simulink model "GPS_Constellation"  (R2018a)
settings: Solver=ode4  StartTime=0  StopTime=time_end  FixedStep=time_step  RelTol=1e-15  AbsTol=1e-15
values from neighbouring files (symbols this model uses):
  c = 299792458    [FFNAV_GPS_Params.mat]    (also in FFNAV_RunGPS.m; Test_GPS_Relativistic.m; Test_Klobuchar_Paper.m)
  GPS_COE = [4.6796815102 2.82369838363 0.203784643463 0.729652347089 1.65659671282 1.15813067845 3.02528391224 5.41010180216 3.56703411206 1.95260455396 0.205879038565 5.92829005708 ... (162 elements, 27x6)]    [FFNAV_GPS_Params.mat]    (also in FFNAV_RunGPS.m = [  268.126*deg2rad    SMA_GPS   ECC_GPS   INC_GPS   357.734*)
  mu = 398600441800000    [FFNAV_GPS_Params.mat]    (also in FFNAV_RunGPS.m; Test_GPS_Relativistic.m = 398600500000000)
undefined symbols (not defined in the file or in its folder): COE_chaser, COE_target
libraries: dspmtrx3 x27
(part 1 of 3)
settings Model: Creator=Cory  LastModifiedBy=Cory
settings SolverCC: AutoScaleAbsTol=off

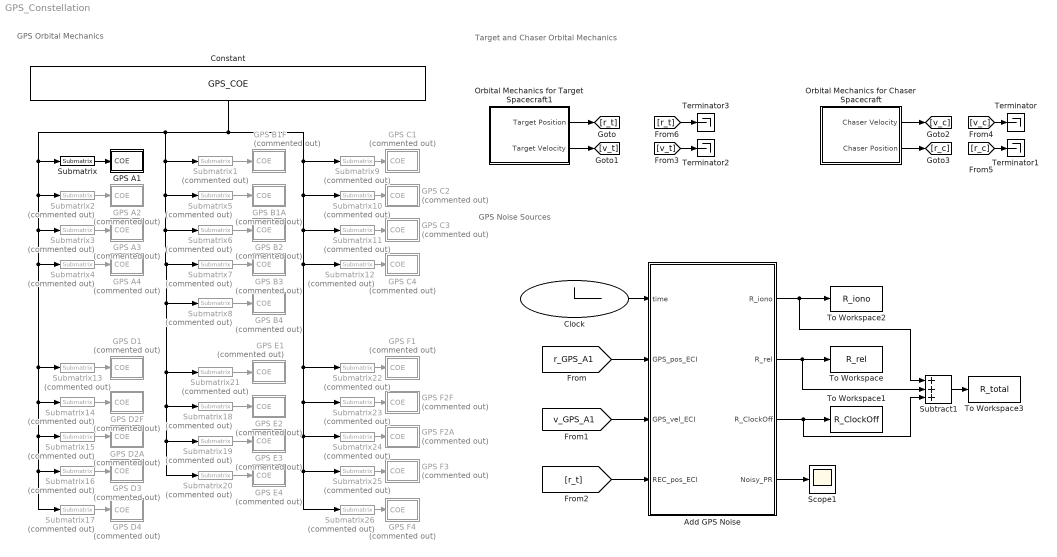
== system GPS_Constellation ==
  note: GPS Noise Sources
  note: GPS Orbital Mechanics
  note: Target and Chaser Orbital Mechanics
  Add GPS Noise : MATLAB Function  TreatAsAtomicUnit=on
  Clock : Clock
      settings: Decimation=1000
  Constant : Constant  Value=GPS_COE
  "GPS A1 " : Subsystem
      mask Display: image('C:\Users\Cory\OneDrive\FFNAV Project\MATLAB Code\NERM EKF Simulation\Masks\GPS Image.jpg');
  GPS A2 : Subsystem  Commented=on
      mask Display: image('C:\Users\Cory\OneDrive\FFNAV Project\MATLAB Code\NERM EKF Simulation\Masks\GPS Image.jpg');
  GPS A3 : Subsystem  Commented=on
      mask Display: image('C:\Users\Cory\OneDrive\FFNAV Project\MATLAB Code\NERM EKF Simulation\Masks\GPS Image.jpg');
  GPS A4 : Subsystem  Commented=on
      mask Display: image('C:\Users\Cory\OneDrive\FFNAV Project\MATLAB Code\NERM EKF Simulation\Masks\GPS Image.jpg');
  GPS B1A : Subsystem  Commented=on
      mask Display: image('C:\Users\Cory\OneDrive\FFNAV Project\MATLAB Code\NERM EKF Simulation\Masks\GPS Image.jpg');
  GPS B1F : Subsystem  Commented=on
      mask Display: image('C:\Users\Cory\OneDrive\FFNAV Project\MATLAB Code\NERM EKF Simulation\Masks\GPS Image.jpg');
  GPS B2 : Subsystem  Commented=on
      mask Display: image('C:\Users\Cory\OneDrive\FFNAV Project\MATLAB Code\NERM EKF Simulation\Masks\GPS Image.jpg');
  GPS B3 : Subsystem  Commented=on
      mask Display: image('C:\Users\Cory\OneDrive\FFNAV Project\MATLAB Code\NERM EKF Simulation\Masks\GPS Image.jpg');
  GPS B4 : Subsystem  Commented=on
      mask Display: image('C:\Users\Cory\OneDrive\FFNAV Project\MATLAB Code\NERM EKF Simulation\Masks\GPS Image.jpg');
  GPS C1 : Subsystem  Commented=on
      mask Display: image('C:\Users\Cory\OneDrive\FFNAV Project\MATLAB Code\NERM EKF Simulation\Masks\GPS Image.jpg');
  GPS C2 : Subsystem  Commented=on
      mask Display: image('C:\Users\Cory\OneDrive\FFNAV Project\MATLAB Code\NERM EKF Simulation\Masks\GPS Image.jpg');
  GPS C3 : Subsystem  Commented=on
      mask Display: image('C:\Users\Cory\OneDrive\FFNAV Project\MATLAB Code\NERM EKF Simulation\Masks\GPS Image.jpg');
  GPS C4 : Subsystem  Commented=on
      mask Display: image('C:\Users\Cory\OneDrive\FFNAV Project\MATLAB Code\NERM EKF Simulation\Masks\GPS Image.jpg');
  GPS D1 : Subsystem  Commented=on
      mask Display: image('C:\Users\Cory\OneDrive\FFNAV Project\MATLAB Code\NERM EKF Simulation\Masks\GPS Image.jpg');
  GPS D2A : Subsystem  Commented=on
      mask Display: image('C:\Users\Cory\OneDrive\FFNAV Project\MATLAB Code\NERM EKF Simulation\Masks\GPS Image.jpg');
  GPS D2F : Subsystem  Commented=on
      mask Display: image('C:\Users\Cory\OneDrive\FFNAV Project\MATLAB Code\NERM EKF Simulation\Masks\GPS Image.jpg');
  GPS D3 : Subsystem  Commented=on
      mask Display: image('C:\Users\Cory\OneDrive\FFNAV Project\MATLAB Code\NERM EKF Simulation\Masks\GPS Image.jpg');
  GPS D4 : Subsystem  Commented=on
      mask Display: image('C:\Users\Cory\OneDrive\FFNAV Project\MATLAB Code\NERM EKF Simulation\Masks\GPS Image.jpg');
  GPS E1 : Subsystem  Commented=on
      mask Display: image('C:\Users\Cory\OneDrive\FFNAV Project\MATLAB Code\NERM EKF Simulation\Masks\GPS Image.jpg');
  GPS E2 : Subsystem  Commented=on
      mask Display: image('C:\Users\Cory\OneDrive\FFNAV Project\MATLAB Code\NERM EKF Simulation\Masks\GPS Image.jpg');
  GPS E3 : Subsystem  Commented=on
      mask Display: image('C:\Users\Cory\OneDrive\FFNAV Project\MATLAB Code\NERM EKF Simulation\Masks\GPS Image.jpg');
  GPS E4 : Subsystem  Commented=on
      mask Display: image('C:\Users\Cory\OneDrive\FFNAV Project\MATLAB Code\NERM EKF Simulation\Masks\GPS Image.jpg');
  GPS F1 : Subsystem  Commented=on
      mask Display: image('C:\Users\Cory\OneDrive\FFNAV Project\MATLAB Code\NERM EKF Simulation\Masks\GPS Image.jpg');
  GPS F2A : Subsystem  Commented=on
      mask Display: image('C:\Users\Cory\OneDrive\FFNAV Project\MATLAB Code\NERM EKF Simulation\Masks\GPS Image.jpg');
  GPS F2F : Subsystem  Commented=on
      mask Display: image('C:\Users\Cory\OneDrive\FFNAV Project\MATLAB Code\NERM EKF Simulation\Masks\GPS Image.jpg');
  GPS F3 : Subsystem  Commented=on
      mask Display: image('C:\Users\Cory\OneDrive\FFNAV Project\MATLAB Code\NERM EKF Simulation\Masks\GPS Image.jpg');
  GPS F4 : Subsystem  Commented=on
      mask Display: image('C:\Users\Cory\OneDrive\FFNAV Project\MATLAB Code\NERM EKF Simulation\Masks\GPS Image.jpg');
  Orbital Mechanics for Target Spacecraft1 : Subsystem
  Orbital Mechanics for Chaser Spacecraft : Subsystem
  Scope1 : Scope
  Submatrix : dspmtrx3/Submatrix  RowSpan=One row  RowStartMode=Index  RowStartIndex=1  RowEndMode=Last  RowEndIndex=1  ColSpan=All columns  ColStartMode=First  ColStartIndex=1  ColEndMode=Last  ColEndIndex=1
  Submatrix1 : dspmtrx3/Submatrix  Commented=on  RowSpan=One row  RowStartMode=Index  RowStartIndex=5  RowEndMode=Last  RowEndIndex=1  ColSpan=All columns  ColStartMode=First  ColStartIndex=1  ColEndMode=Last  ColEndIndex=1
  Submatrix10 : dspmtrx3/Submatrix  Commented=on  RowSpan=One row  RowStartMode=Index  RowStartIndex=11  RowEndMode=Last  RowEndIndex=1  ColSpan=All columns  ColStartMode=First  ColStartIndex=1  ColEndMode=Last  ColEndIndex=1
  Submatrix11 : dspmtrx3/Submatrix  Commented=on  RowSpan=One row  RowStartMode=Index  RowStartIndex=12  RowEndMode=Last  RowEndIndex=1  ColSpan=All columns  ColStartMode=First  ColStartIndex=1  ColEndMode=Last  ColEndIndex=1
  Submatrix12 : dspmtrx3/Submatrix  Commented=on  RowSpan=One row  RowStartMode=Index  RowStartIndex=13  RowEndMode=Last  RowEndIndex=1  ColSpan=All columns  ColStartMode=First  ColStartIndex=1  ColEndMode=Last  ColEndIndex=1
  Submatrix13 : dspmtrx3/Submatrix  Commented=on  RowSpan=One row  RowStartMode=Index  RowStartIndex=14  RowEndMode=Last  RowEndIndex=1  ColSpan=All columns  ColStartMode=First  ColStartIndex=1  ColEndMode=Last  ColEndIndex=1
  Submatrix14 : dspmtrx3/Submatrix  Commented=on  RowSpan=One row  RowStartMode=Index  RowStartIndex=15  RowEndMode=Last  RowEndIndex=1  ColSpan=All columns  ColStartMode=First  ColStartIndex=1  ColEndMode=Last  ColEndIndex=1
  Submatrix15 : dspmtrx3/Submatrix  Commented=on  RowSpan=One row  RowStartMode=Index  RowStartIndex=16  RowEndMode=Last  RowEndIndex=1  ColSpan=All columns  ColStartMode=First  ColStartIndex=1  ColEndMode=Last  ColEndIndex=1
  Submatrix16 : dspmtrx3/Submatrix  Commented=on  RowSpan=One row  RowStartMode=Index  RowStartIndex=17  RowEndMode=Last  RowEndIndex=1  ColSpan=All columns  ColStartMode=First  ColStartIndex=1  ColEndMode=Last  ColEndIndex=1
  Submatrix17 : dspmtrx3/Submatrix  Commented=on  RowSpan=One row  RowStartMode=Index  RowStartIndex=18  RowEndMode=Last  RowEndIndex=1  ColSpan=All columns  ColStartMode=First  ColStartIndex=1  ColEndMode=Last  ColEndIndex=1
  Submatrix18 : dspmtrx3/Submatrix  Commented=on  RowSpan=One row  RowStartMode=Index  RowStartIndex=20  RowEndMode=Last  RowEndIndex=1  ColSpan=All columns  ColStartMode=First  ColStartIndex=1  ColEndMode=Last  ColEndIndex=1
  Submatrix19 : dspmtrx3/Submatrix  Commented=on  RowSpan=One row  RowStartMode=Index  RowStartIndex=21  RowEndMode=Last  RowEndIndex=1  ColSpan=All columns  ColStartMode=First  ColStartIndex=1  ColEndMode=Last  ColEndIndex=1
  Submatrix2 : dspmtrx3/Submatrix  Commented=on  RowSpan=One row  RowStartMode=Index  RowStartIndex=2  RowEndMode=Last  RowEndIndex=1  ColSpan=All columns  ColStartMode=First  ColStartIndex=1  ColEndMode=Last  ColEndIndex=1
  Submatrix20 : dspmtrx3/Submatrix  Commented=on  RowSpan=One row  RowStartMode=Index  RowStartIndex=22  RowEndMode=Last  RowEndIndex=1  ColSpan=All columns  ColStartMode=First  ColStartIndex=1  ColEndMode=Last  ColEndIndex=1
  Submatrix21 : dspmtrx3/Submatrix  Commented=on  RowSpan=One row  RowStartMode=Index  RowStartIndex=19  RowEndMode=Last  RowEndIndex=1  ColSpan=All columns  ColStartMode=First  ColStartIndex=1  ColEndMode=Last  ColEndIndex=1
  Submatrix22 : dspmtrx3/Submatrix  Commented=on  RowSpan=One row  RowStartMode=Index  RowStartIndex=23  RowEndMode=Last  RowEndIndex=1  ColSpan=All columns  ColStartMode=First  ColStartIndex=1  ColEndMode=Last  ColEndIndex=1
  Submatrix23 : dspmtrx3/Submatrix  Commented=on  RowSpan=One row  RowStartMode=Index  RowStartIndex=24  RowEndMode=Last  RowEndIndex=1  ColSpan=All columns  ColStartMode=First  ColStartIndex=1  ColEndMode=Last  ColEndIndex=1
  Submatrix24 : dspmtrx3/Submatrix  Commented=on  RowSpan=One row  RowStartMode=Index  RowStartIndex=25  RowEndMode=Last  RowEndIndex=1  ColSpan=All columns  ColStartMode=First  ColStartIndex=1  ColEndMode=Last  ColEndIndex=1
  Submatrix25 : dspmtrx3/Submatrix  Commented=on  RowSpan=One row  RowStartMode=Index  RowStartIndex=26  RowEndMode=Last  RowEndIndex=1  ColSpan=All columns  ColStartMode=First  ColStartIndex=1  ColEndMode=Last  ColEndIndex=1
  Submatrix26 : dspmtrx3/Submatrix  Commented=on  RowSpan=One row  RowStartMode=Index  RowStartIndex=27  RowEndMode=Last  RowEndIndex=1  ColSpan=All columns  ColStartMode=First  ColStartIndex=1  ColEndMode=Last  ColEndIndex=1
  Submatrix3 : dspmtrx3/Submatrix  Commented=on  RowSpan=One row  RowStartMode=Index  RowStartIndex=3  RowEndMode=Last  RowEndIndex=1  ColSpan=All columns  ColStartMode=First  ColStartIndex=1  ColEndMode=Last  ColEndIndex=1
  Submatrix4 : dspmtrx3/Submatrix  Commented=on  RowSpan=One row  RowStartMode=Index  RowStartIndex=4  RowEndMode=Last  RowEndIndex=1  ColSpan=All columns  ColStartMode=First  ColStartIndex=1  ColEndMode=Last  ColEndIndex=1
  Submatrix5 : dspmtrx3/Submatrix  Commented=on  RowSpan=One row  RowStartMode=Index  RowStartIndex=6  RowEndMode=Last  RowEndIndex=1  ColSpan=All columns  ColStartMode=First  ColStartIndex=1  ColEndMode=Last  ColEndIndex=1
  Submatrix6 : dspmtrx3/Submatrix  Commented=on  RowSpan=One row  RowStartMode=Index  RowStartIndex=7  RowEndMode=Last  RowEndIndex=1  ColSpan=All columns  ColStartMode=First  ColStartIndex=1  ColEndMode=Last  ColEndIndex=1
  Submatrix7 : dspmtrx3/Submatrix  Commented=on  RowSpan=One row  RowStartMode=Index  RowStartIndex=8  RowEndMode=Last  RowEndIndex=1  ColSpan=All columns  ColStartMode=First  ColStartIndex=1  ColEndMode=Last  ColEndIndex=1
  Submatrix8 : dspmtrx3/Submatrix  Commented=on  RowSpan=One row  RowStartMode=Index  RowStartIndex=9  RowEndMode=Last  RowEndIndex=1  ColSpan=All columns  ColStartMode=First  ColStartIndex=1  ColEndMode=Last  ColEndIndex=1
  Submatrix9 : dspmtrx3/Submatrix  Commented=on  RowSpan=One row  RowStartMode=Index  RowStartIndex=10  RowEndMode=Last  RowEndIndex=1  ColSpan=All columns  ColStartMode=First  ColStartIndex=1  ColEndMode=Last  ColEndIndex=1
  Subtract1 : Sum  Inputs=+++
  Terminator{,1..3} (4 alike) : Terminator
  To Workspace : ToWorkspace  VariableName=R_rel  SampleTime=-1
      settings: Save2DSignal=2-D array (concatenate along first dimension)
  To Workspace1 : ToWorkspace  VariableName=R_ClockOff  SampleTime=-1
      settings: Save2DSignal=2-D array (concatenate along first dimension)
  To Workspace2 : ToWorkspace  VariableName=R_iono  SampleTime=-1
      settings: Save2DSignal=2-D array (concatenate along first dimension)
  To Workspace3 : ToWorkspace  VariableName=R_total  SampleTime=-1
      settings: Save2DSignal=2-D array (concatenate along first dimension)
  wires:
  Submatrix/1 -> "GPS A1 "/1(COE)
  Submatrix1/1 -> GPS B1F/1(COE)
  Submatrix2/1 -> GPS A2/1(COE)
  Submatrix3/1 -> GPS A3/1(COE)
  Submatrix4/1 -> GPS A4/1(COE)
  Submatrix5/1 -> GPS B1A/1(COE)
  Submatrix6/1 -> GPS B2/1(COE)
  Submatrix7/1 -> GPS B3/1(COE)
  Submatrix8/1 -> GPS B4/1(COE)
  Submatrix10/1 -> GPS C2/1(COE)
  Submatrix11/1 -> GPS C3/1(COE)
  Submatrix12/1 -> GPS C4/1(COE)
  Submatrix9/1 -> GPS C1/1(COE)
  Submatrix14/1 -> GPS D2F/1(COE)
  Submatrix15/1 -> GPS D2A/1(COE)
  Submatrix17/1 -> GPS D4/1(COE)
  Submatrix16/1 -> GPS D3/1(COE)
  Submatrix13/1 -> GPS D1/1(COE)
  Submatrix19/1 -> GPS E3/1(COE)
  Submatrix18/1 -> GPS E2/1(COE)
  Submatrix21/1 -> GPS E1/1(COE)
  Submatrix20/1 -> GPS E4/1(COE)
  Submatrix23/1 -> GPS F2F/1(COE)
  Constant/1 -> Submatrix17/1, Submatrix16/1, Submatrix15/1, Submatrix14/1, Submatrix13/1, Submatrix4/1, Submatrix3/1, Submatrix2/1, Submatrix/1, Submatrix8/1, Submatrix21/1, Submatrix18/1, Submatrix19/1, Submatrix20/1, Submatrix7/1, Submatrix6/1, Submatrix5/1, Submatrix1/1, Submatrix12/1, Submatrix22/1, Submatrix23/1, Submatrix24/1, Submatrix25/1, Submatrix26/1, Submatrix11/1, Submatrix10/1, Submatrix9/1
  Submatrix26/1 -> GPS F4/1(COE)
  Submatrix24/1 -> GPS F2A/1(COE)
  Submatrix25/1 -> GPS F3/1(COE)
  Submatrix22/1 -> GPS F1/1(COE)
  Clock/1 -> Add GPS Noise/1(time)
  Add GPS Noise/1(R_iono) -> Subtract1/1, To Workspace2/1
  Add GPS Noise/4(Noisy_PR) -> Scope1/1
  [r_GPS_A1] -> Add GPS Noise/2(GPS_pos_ECI)
  [v_GPS_A1] -> Add GPS Noise/3(GPS_vel_ECI)
  [r_t] -> Add GPS Noise/4(REC_pos_ECI)
  Add GPS Noise/2(R_rel) -> Subtract1/2, To Workspace/1
  Add GPS Noise/3(R_ClockOff) -> Subtract1/3, To Workspace1/1
  Subtract1/1 -> To Workspace3/1
  Orbital Mechanics for Chaser Spacecraft/2(Chaser Position) -> [r_c]
  Orbital Mechanics for Target Spacecraft1/1(Target Position) -> [r_t]
  Orbital Mechanics for Target Spacecraft1/2(Target Velocity) -> [v_t]
  Orbital Mechanics for Chaser Spacecraft/1(Chaser Velocity) -> [v_c]
  [v_c] -> Terminator/1
  [r_c] -> Terminator1/1
  [v_t] -> Terminator2/1
  [r_t] -> Terminator3/1

== system GPS_Constellation/GPS A1  ==
  COE : Inport
  Mux : Mux  Inputs=2
  Orbital Mechanics : Subsystem
  To Workspace : ToWorkspace  VariableName=GPS_A1  SampleTime=-1
      settings: Save2DSignal=2-D array (concatenate along first dimension)
  tag scope: r_GPS_A1=global, v_GPS_A1=global
  wires:
  Orbital Mechanics/2(Velocity (v)) -> [v_GPS_A1], Mux/2
  COE/1 -> Orbital Mechanics/1(COE)
  Mux/1 -> To Workspace/1
  Orbital Mechanics/1(Position (r)) -> Mux/1, [r_GPS_A1]

== system GPS_Constellation/GPS A2 ==
  COE : Inport
  Mux : Mux  Inputs=2
  Orbital Mechanics1 : Subsystem
  To Workspace : ToWorkspace  VariableName=GPS_A2  SampleTime=-1
      settings: Save2DSignal=2-D array (concatenate along first dimension)
  wires:
  Orbital Mechanics1/2(Velocity (v)) -> Mux/2
  COE/1 -> Orbital Mechanics1/1(COE)
  Orbital Mechanics1/1(Position (r)) -> Mux/1
  Mux/1 -> To Workspace/1

== system GPS_Constellation/GPS A3 ==
  COE : Inport
  Mux : Mux  Inputs=2
  Orbital Mechanics : Subsystem
  To Workspace : ToWorkspace  VariableName=GPS_A3  SampleTime=-1
      settings: Save2DSignal=2-D array (concatenate along first dimension)
  wires:
  Orbital Mechanics/2(Velocity (v)) -> Mux/2
  COE/1 -> Orbital Mechanics/1(COE)
  Orbital Mechanics/1(Position (r)) -> Mux/1
  Mux/1 -> To Workspace/1

== system GPS_Constellation/GPS A4 ==
  COE : Inport
  Mux : Mux  Inputs=2
  Orbital Mechanics : Subsystem
  To Workspace : ToWorkspace  VariableName=GPS_A4  SampleTime=-1
      settings: Save2DSignal=2-D array (concatenate along first dimension)
  wires:
  Orbital Mechanics/2(Velocity (v)) -> Mux/2
  COE/1 -> Orbital Mechanics/1(COE)
  Orbital Mechanics/1(Position (r)) -> Mux/1
  Mux/1 -> To Workspace/1

== system GPS_Constellation/GPS B1A ==
  COE : Inport
  Mux : Mux  Inputs=2
  Orbital Mechanics : Subsystem
  To Workspace : ToWorkspace  VariableName=GPS_B1A  SampleTime=-1
      settings: Save2DSignal=2-D array (concatenate along first dimension)
  wires:
  Orbital Mechanics/2(Velocity (v)) -> Mux/2
  COE/1 -> Orbital Mechanics/1(COE)
  Orbital Mechanics/1(Position (r)) -> Mux/1
  Mux/1 -> To Workspace/1

== system GPS_Constellation/GPS B1F ==
  COE : Inport
  Mux : Mux  Inputs=2
  Orbital Mechanics : Subsystem
  To Workspace : ToWorkspace  VariableName=GPS_B1F  SampleTime=-1
      settings: Save2DSignal=2-D array (concatenate along first dimension)
  wires:
  Orbital Mechanics/2(Velocity (v)) -> Mux/2
  COE/1 -> Orbital Mechanics/1(COE)
  Orbital Mechanics/1(Position (r)) -> Mux/1
  Mux/1 -> To Workspace/1

== system GPS_Constellation/GPS B2 ==
  COE : Inport
  Mux : Mux  Inputs=2
  Orbital Mechanics : Subsystem
  To Workspace : ToWorkspace  VariableName=GPS_B2  SampleTime=-1
      settings: Save2DSignal=2-D array (concatenate along first dimension)
  wires:
  Orbital Mechanics/2(Velocity (v)) -> Mux/2
  COE/1 -> Orbital Mechanics/1(COE)
  Orbital Mechanics/1(Position (r)) -> Mux/1
  Mux/1 -> To Workspace/1

== system GPS_Constellation/GPS B3 ==
  COE : Inport
  Mux : Mux  Inputs=2
  Orbital Mechanics : Subsystem
  To Workspace : ToWorkspace  VariableName=GPS_B3  SampleTime=-1
      settings: Save2DSignal=2-D array (concatenate along first dimension)
  wires:
  Orbital Mechanics/2(Velocity (v)) -> Mux/2
  COE/1 -> Orbital Mechanics/1(COE)
  Orbital Mechanics/1(Position (r)) -> Mux/1
  Mux/1 -> To Workspace/1

== system GPS_Constellation/GPS B4 ==
  COE : Inport
  Mux : Mux  Inputs=2
  Orbital Mechanics : Subsystem
  To Workspace : ToWorkspace  VariableName=GPS_B4  SampleTime=-1
      settings: Save2DSignal=2-D array (concatenate along first dimension)
  wires:
  Orbital Mechanics/2(Velocity (v)) -> Mux/2
  COE/1 -> Orbital Mechanics/1(COE)
  Orbital Mechanics/1(Position (r)) -> Mux/1
  Mux/1 -> To Workspace/1

== system GPS_Constellation/GPS C1 ==
  COE : Inport
  Mux : Mux  Inputs=2
  Orbital Mechanics : Subsystem
  To Workspace : ToWorkspace  VariableName=GPS_C1  SampleTime=-1
      settings: Save2DSignal=2-D array (concatenate along first dimension)
  wires:
  Orbital Mechanics/2(Velocity (v)) -> Mux/2
  COE/1 -> Orbital Mechanics/1(COE)
  Orbital Mechanics/1(Position (r)) -> Mux/1
  Mux/1 -> To Workspace/1

== system GPS_Constellation/GPS C2 ==
  COE : Inport
  Mux : Mux  Inputs=2
  Orbital Mechanics : Subsystem
  To Workspace : ToWorkspace  VariableName=GPS_C2  SampleTime=-1
      settings: Save2DSignal=2-D array (concatenate along first dimension)
  wires:
  Orbital Mechanics/2(Velocity (v)) -> Mux/2
  COE/1 -> Orbital Mechanics/1(COE)
  Orbital Mechanics/1(Position (r)) -> Mux/1
  Mux/1 -> To Workspace/1

== system GPS_Constellation/GPS C3 ==
  COE : Inport
  Mux : Mux  Inputs=2
  Orbital Mechanics : Subsystem
  To Workspace : ToWorkspace  VariableName=GPS_C3  SampleTime=-1
      settings: Save2DSignal=2-D array (concatenate along first dimension)
  wires:
  Orbital Mechanics/2(Velocity (v)) -> Mux/2
  COE/1 -> Orbital Mechanics/1(COE)
  Orbital Mechanics/1(Position (r)) -> Mux/1
  Mux/1 -> To Workspace/1

== system GPS_Constellation/GPS C4 ==
  COE : Inport
  Mux : Mux  Inputs=2
  Orbital Mechanics : Subsystem
  To Workspace : ToWorkspace  VariableName=GPS_C4  SampleTime=-1
      settings: Save2DSignal=2-D array (concatenate along first dimension)
  wires:
  Orbital Mechanics/2(Velocity (v)) -> Mux/2
  COE/1 -> Orbital Mechanics/1(COE)
  Orbital Mechanics/1(Position (r)) -> Mux/1
  Mux/1 -> To Workspace/1

== system GPS_Constellation/GPS D1 ==
  COE : Inport
  Mux : Mux  Inputs=2
  Orbital Mechanics : Subsystem
  To Workspace : ToWorkspace  VariableName=GPS_D1  SampleTime=-1
      settings: Save2DSignal=2-D array (concatenate along first dimension)
  wires:
  Orbital Mechanics/2(Velocity (v)) -> Mux/2
  COE/1 -> Orbital Mechanics/1(COE)
  Orbital Mechanics/1(Position (r)) -> Mux/1
  Mux/1 -> To Workspace/1

== system GPS_Constellation/GPS D2A ==
  COE : Inport
  Mux : Mux  Inputs=2
  Orbital Mechanics : Subsystem
  To Workspace : ToWorkspace  VariableName=GPS_D2A  SampleTime=-1
      settings: Save2DSignal=2-D array (concatenate along first dimension)
  wires:
  Orbital Mechanics/2(Velocity (v)) -> Mux/2
  COE/1 -> Orbital Mechanics/1(COE)
  Orbital Mechanics/1(Position (r)) -> Mux/1
  Mux/1 -> To Workspace/1

== system GPS_Constellation/GPS D2F ==
  COE : Inport
  Mux : Mux  Inputs=2
  Orbital Mechanics : Subsystem
  To Workspace : ToWorkspace  VariableName=GPS_D2F  SampleTime=-1
      settings: Save2DSignal=2-D array (concatenate along first dimension)
  wires:
  Orbital Mechanics/2(Velocity (v)) -> Mux/2
  COE/1 -> Orbital Mechanics/1(COE)
  Orbital Mechanics/1(Position (r)) -> Mux/1
  Mux/1 -> To Workspace/1

== system GPS_Constellation/GPS D3 ==
  COE : Inport
  Mux : Mux  Inputs=2
  Orbital Mechanics : Subsystem
  To Workspace : ToWorkspace  VariableName=GPS_D3  SampleTime=-1
      settings: Save2DSignal=2-D array (concatenate along first dimension)
  wires:
  Orbital Mechanics/2(Velocity (v)) -> Mux/2
  COE/1 -> Orbital Mechanics/1(COE)
  Orbital Mechanics/1(Position (r)) -> Mux/1
  Mux/1 -> To Workspace/1

== system GPS_Constellation/GPS D4 ==
  COE : Inport
  Mux : Mux  Inputs=2
  Orbital Mechanics : Subsystem
  To Workspace : ToWorkspace  VariableName=GPS_D4  SampleTime=-1
      settings: Save2DSignal=2-D array (concatenate along first dimension)
  wires:
  Orbital Mechanics/2(Velocity (v)) -> Mux/2
  COE/1 -> Orbital Mechanics/1(COE)
  Orbital Mechanics/1(Position (r)) -> Mux/1
  Mux/1 -> To Workspace/1

== system GPS_Constellation/GPS E1 ==
  COE : Inport
  Mux : Mux  Inputs=2
  Orbital Mechanics : Subsystem
  To Workspace : ToWorkspace  VariableName=GPS_E1  SampleTime=-1
      settings: Save2DSignal=2-D array (concatenate along first dimension)
  wires:
  Orbital Mechanics/2(Velocity (v)) -> Mux/2
  COE/1 -> Orbital Mechanics/1(COE)
  Orbital Mechanics/1(Position (r)) -> Mux/1
  Mux/1 -> To Workspace/1

== system GPS_Constellation/GPS E2 ==
  COE : Inport
  Mux : Mux  Inputs=2
  Orbital Mechanics : Subsystem
  To Workspace : ToWorkspace  VariableName=GPS_E2  SampleTime=-1
      settings: Save2DSignal=2-D array (concatenate along first dimension)
  wires:
  Orbital Mechanics/2(Velocity (v)) -> Mux/2
  COE/1 -> Orbital Mechanics/1(COE)
  Orbital Mechanics/1(Position (r)) -> Mux/1
  Mux/1 -> To Workspace/1

== system GPS_Constellation/GPS E3 ==
  COE : Inport
  Mux : Mux  Inputs=2
  Orbital Mechanics : Subsystem
  To Workspace : ToWorkspace  VariableName=GPS_E3  SampleTime=-1
      settings: Save2DSignal=2-D array (concatenate along first dimension)
  wires:
  Orbital Mechanics/2(Velocity (v)) -> Mux/2
  COE/1 -> Orbital Mechanics/1(COE)
  Orbital Mechanics/1(Position (r)) -> Mux/1
  Mux/1 -> To Workspace/1

== system GPS_Constellation/GPS E4 ==
  COE : Inport
  Mux : Mux  Inputs=2
  Orbital Mechanics : Subsystem
  To Workspace : ToWorkspace  VariableName=GPS_E4  SampleTime=-1
      settings: Save2DSignal=2-D array (concatenate along first dimension)
  wires:
  Orbital Mechanics/2(Velocity (v)) -> Mux/2
  COE/1 -> Orbital Mechanics/1(COE)
  Orbital Mechanics/1(Position (r)) -> Mux/1
  Mux/1 -> To Workspace/1

== system GPS_Constellation/GPS F1 ==
  COE : Inport
  Mux : Mux  Inputs=2
  Orbital Mechanics : Subsystem
  To Workspace : ToWorkspace  VariableName=GPS_F1  SampleTime=-1
      settings: Save2DSignal=2-D array (concatenate along first dimension)
  wires:
  Orbital Mechanics/2(Velocity (v)) -> Mux/2
  COE/1 -> Orbital Mechanics/1(COE)
  Orbital Mechanics/1(Position (r)) -> Mux/1
  Mux/1 -> To Workspace/1

== system GPS_Constellation/GPS F2A ==
  COE : Inport
  Mux : Mux  Inputs=2
  Orbital Mechanics : Subsystem
  To Workspace : ToWorkspace  VariableName=GPS_F2A  SampleTime=-1
      settings: Save2DSignal=2-D array (concatenate along first dimension)
  wires:
  Orbital Mechanics/2(Velocity (v)) -> Mux/2
  COE/1 -> Orbital Mechanics/1(COE)
  Orbital Mechanics/1(Position (r)) -> Mux/1
  Mux/1 -> To Workspace/1

== system GPS_Constellation/GPS F2F ==
  COE : Inport
  Mux : Mux  Inputs=2
  Orbital Mechanics : Subsystem
  To Workspace : ToWorkspace  VariableName=GPS_F2F  SampleTime=-1
      settings: Save2DSignal=2-D array (concatenate along first dimension)
  wires:
  Orbital Mechanics/2(Velocity (v)) -> Mux/2
  COE/1 -> Orbital Mechanics/1(COE)
  Orbital Mechanics/1(Position (r)) -> Mux/1
  Mux/1 -> To Workspace/1

== system GPS_Constellation/GPS F3 ==
  COE : Inport
  Mux : Mux  Inputs=2
  Orbital Mechanics : Subsystem
  To Workspace : ToWorkspace  VariableName=GPS_F3  SampleTime=-1
      settings: Save2DSignal=2-D array (concatenate along first dimension)
  wires:
  Orbital Mechanics/2(Velocity (v)) -> Mux/2
  COE/1 -> Orbital Mechanics/1(COE)
  Orbital Mechanics/1(Position (r)) -> Mux/1
  Mux/1 -> To Workspace/1

== system GPS_Constellation/GPS F4 ==
  COE : Inport
  Mux : Mux  Inputs=2
  Orbital Mechanics : Subsystem
  To Workspace : ToWorkspace  VariableName=GPS_F4  SampleTime=-1
      settings: Save2DSignal=2-D array (concatenate along first dimension)
  wires:
  Orbital Mechanics/2(Velocity (v)) -> Mux/2
  COE/1 -> Orbital Mechanics/1(COE)
  Orbital Mechanics/1(Position (r)) -> Mux/1
  Mux/1 -> To Workspace/1

== system GPS_Constellation/Orbital Mechanics for Target Spacecraft1 ==
  Integrator : Integrator  InitialConditionSource=external
  Integrator1 : Integrator  InitialConditionSource=external
  MATLAB Function1 : MATLAB Function  TreatAsAtomicUnit=on
  Target Orbital Mechanics : MATLAB Function  TreatAsAtomicUnit=on
  To Workspace1 : ToWorkspace  VariableName=r_target_ECI  SampleTime=-1
  To Workspace2 : ToWorkspace  VariableName=v_target_ECI  SampleTime=-1
  Target Position : Outport
  Target Velocity : Outport  Port=2
  wires:
  Integrator/1 -> To Workspace2/1, Target Velocity/1, Integrator1/1  "r_dot"
  MATLAB Function1/1(r_ddot) -> Integrator/1  "r_ddot"
  Integrator1/1 -> MATLAB Function1/1(r), To Workspace1/1, Target Position/1  "getr"
  Target Orbital Mechanics/2(r_ECI) -> Integrator1/2
  Target Orbital Mechanics/1(v_ECI) -> Integrator/2  "V0"

== system GPS_Constellation/Orbital Mechanics for Chaser Spacecraft ==
  Integrator : Integrator  InitialConditionSource=external
  Integrator1 : Integrator  InitialConditionSource=external
  MATLAB Function1 : MATLAB Function  TreatAsAtomicUnit=on
  Orbital Mechanics : MATLAB Function  TreatAsAtomicUnit=on
  To Workspace1 : ToWorkspace  VariableName=r_chaser_ECI  SampleTime=-1
  To Workspace2 : ToWorkspace  VariableName=v_chaser_ECI  SampleTime=-1
  Chaser Velocity : Outport
  Chaser Position : Outport  Port=2
  wires:
  Integrator/1 -> To Workspace2/1, Chaser Velocity/1, Integrator1/1  "r_dot"
  MATLAB Function1/1(r_ddot) -> Integrator/1  "r_ddot"
  Integrator1/1 -> To Workspace1/1, MATLAB Function1/1(r), Chaser Position/1  "r"
  Orbital Mechanics/2(r_ECI) -> Integrator1/2
  Orbital Mechanics/1(v_ECI) -> Integrator/2  "V0"

== system GPS_Constellation/GPS A1 /Orbital Mechanics ==
  COE : Inport
  Integrator : Integrator  InitialConditionSource=external
  Integrator1 : Integrator  InitialConditionSource=external
  MATLAB Function1 : MATLAB Function  TreatAsAtomicUnit=on
  Orbital Mechanics : MATLAB Function  TreatAsAtomicUnit=on
  Position (r) : Outport
  Velocity (v) : Outport  Port=2
  wires:
  Integrator/1 -> Velocity (v)/1, Integrator1/1  "r_dot"
  MATLAB Function1/1(r_ddot) -> Integrator/1  "r_ddot"
  Integrator1/1 -> Position (r)/1, MATLAB Function1/1(R_sat)  "r"
  Orbital Mechanics/2(r_ECI) -> Integrator1/2
  Orbital Mechanics/1(v_ECI) -> Integrator/2  "V0"
  COE/1 -> Orbital Mechanics/1(COE)

== system GPS_Constellation/GPS A2/Orbital Mechanics1 ==
  COE : Inport
  Integrator : Integrator  InitialConditionSource=external
  Integrator1 : Integrator  InitialConditionSource=external
  MATLAB Function1 : MATLAB Function  TreatAsAtomicUnit=on
  Orbital Mechanics : MATLAB Function  TreatAsAtomicUnit=on
  Position (r) : Outport
  Velocity (v) : Outport  Port=2
  wires:
  Integrator/1 -> Velocity (v)/1, Integrator1/1  "r_dot"
  MATLAB Function1/1(r_ddot) -> Integrator/1  "r_ddot"
  Integrator1/1 -> Position (r)/1, MATLAB Function1/1(r)  "r"
  Orbital Mechanics/2(r_ECI) -> Integrator1/2
  Orbital Mechanics/1(v_ECI) -> Integrator/2  "V0"
  COE/1 -> Orbital Mechanics/1(COE)

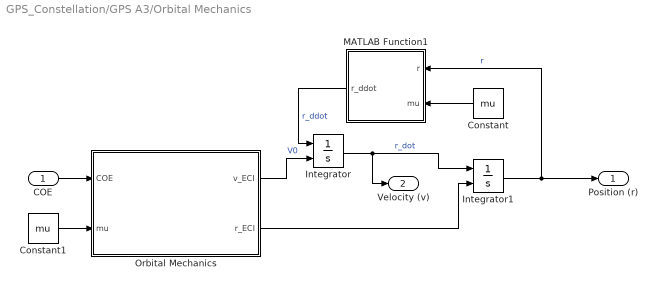
== system GPS_Constellation/GPS A3/Orbital Mechanics ==
  COE : Inport
  Constant : Constant  Value=mu
  Constant1 : Constant  Value=mu
  Integrator : Integrator  InitialConditionSource=external
  Integrator1 : Integrator  InitialConditionSource=external
  MATLAB Function1 : MATLAB Function  TreatAsAtomicUnit=on
  Orbital Mechanics : MATLAB Function  TreatAsAtomicUnit=on
  Position (r) : Outport
  Velocity (v) : Outport  Port=2
  wires:
  Integrator/1 -> Velocity (v)/1, Integrator1/1  "r_dot"
  MATLAB Function1/1(r_ddot) -> Integrator/1  "r_ddot"
  Integrator1/1 -> Position (r)/1, MATLAB Function1/1(r)  "r"
  Orbital Mechanics/2(r_ECI) -> Integrator1/2
  Orbital Mechanics/1(v_ECI) -> Integrator/2  "V0"
  COE/1 -> Orbital Mechanics/1(COE)
  Constant/1 -> MATLAB Function1/2(mu)
  Constant1/1 -> Orbital Mechanics/2(mu)

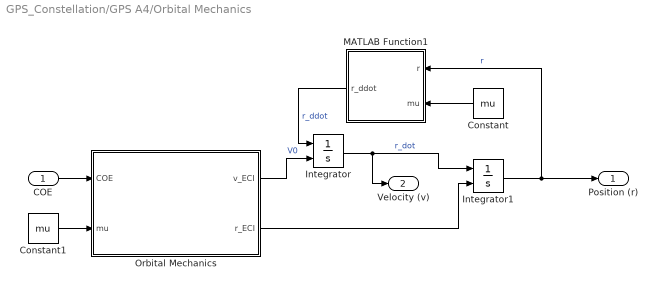
== system GPS_Constellation/GPS A4/Orbital Mechanics ==
  COE : Inport
  Constant : Constant  Value=mu
  Constant1 : Constant  Value=mu
  Integrator : Integrator  InitialConditionSource=external
  Integrator1 : Integrator  InitialConditionSource=external
  MATLAB Function1 : MATLAB Function  TreatAsAtomicUnit=on
  Orbital Mechanics : MATLAB Function  TreatAsAtomicUnit=on
  Position (r) : Outport
  Velocity (v) : Outport  Port=2
  wires:
  Integrator/1 -> Velocity (v)/1, Integrator1/1  "r_dot"
  MATLAB Function1/1(r_ddot) -> Integrator/1  "r_ddot"
  Integrator1/1 -> Position (r)/1, MATLAB Function1/1(r)  "r"
  Orbital Mechanics/2(r_ECI) -> Integrator1/2
  Orbital Mechanics/1(v_ECI) -> Integrator/2  "V0"
  COE/1 -> Orbital Mechanics/1(COE)
  Constant/1 -> MATLAB Function1/2(mu)
  Constant1/1 -> Orbital Mechanics/2(mu)

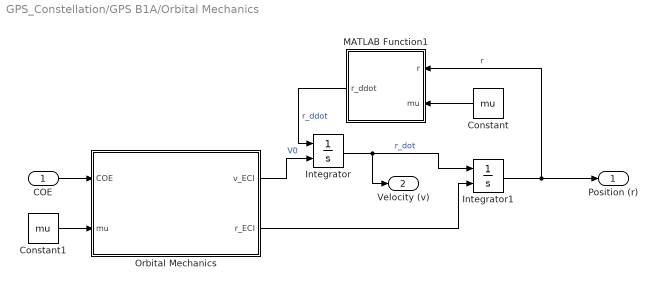
== system GPS_Constellation/GPS B1A/Orbital Mechanics ==
  COE : Inport
  Constant : Constant  Value=mu
  Constant1 : Constant  Value=mu
  Integrator : Integrator  InitialConditionSource=external
  Integrator1 : Integrator  InitialConditionSource=external
  MATLAB Function1 : MATLAB Function  TreatAsAtomicUnit=on
  Orbital Mechanics : MATLAB Function  TreatAsAtomicUnit=on
  Position (r) : Outport
  Velocity (v) : Outport  Port=2
  wires:
  Integrator/1 -> Velocity (v)/1, Integrator1/1  "r_dot"
  MATLAB Function1/1(r_ddot) -> Integrator/1  "r_ddot"
  Integrator1/1 -> Position (r)/1, MATLAB Function1/1(r)  "r"
  Orbital Mechanics/2(r_ECI) -> Integrator1/2
  Orbital Mechanics/1(v_ECI) -> Integrator/2  "V0"
  COE/1 -> Orbital Mechanics/1(COE)
  Constant/1 -> MATLAB Function1/2(mu)
  Constant1/1 -> Orbital Mechanics/2(mu)

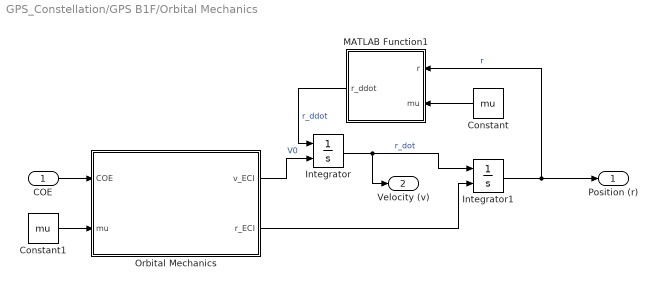
== system GPS_Constellation/GPS B1F/Orbital Mechanics ==
  COE : Inport
  Constant : Constant  Value=mu
  Constant1 : Constant  Value=mu
  Integrator : Integrator  InitialConditionSource=external
  Integrator1 : Integrator  InitialConditionSource=external
  MATLAB Function1 : MATLAB Function  TreatAsAtomicUnit=on
  Orbital Mechanics : MATLAB Function  TreatAsAtomicUnit=on
  Position (r) : Outport
  Velocity (v) : Outport  Port=2
  wires:
  Integrator/1 -> Velocity (v)/1, Integrator1/1  "r_dot"
  MATLAB Function1/1(r_ddot) -> Integrator/1  "r_ddot"
  Integrator1/1 -> Position (r)/1, MATLAB Function1/1(r)  "r"
  Orbital Mechanics/2(r_ECI) -> Integrator1/2
  Orbital Mechanics/1(v_ECI) -> Integrator/2  "V0"
  COE/1 -> Orbital Mechanics/1(COE)
  Constant/1 -> MATLAB Function1/2(mu)
  Constant1/1 -> Orbital Mechanics/2(mu)

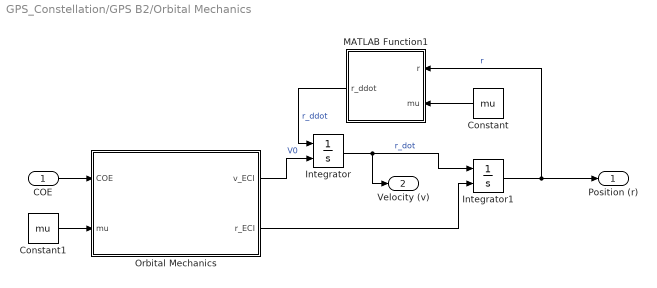
== system GPS_Constellation/GPS B2/Orbital Mechanics ==
  COE : Inport
  Constant : Constant  Value=mu
  Constant1 : Constant  Value=mu
  Integrator : Integrator  InitialConditionSource=external
  Integrator1 : Integrator  InitialConditionSource=external
  MATLAB Function1 : MATLAB Function  TreatAsAtomicUnit=on
  Orbital Mechanics : MATLAB Function  TreatAsAtomicUnit=on
  Position (r) : Outport
  Velocity (v) : Outport  Port=2
  wires:
  Integrator/1 -> Velocity (v)/1, Integrator1/1  "r_dot"
  MATLAB Function1/1(r_ddot) -> Integrator/1  "r_ddot"
  Integrator1/1 -> Position (r)/1, MATLAB Function1/1(r)  "r"
  Orbital Mechanics/2(r_ECI) -> Integrator1/2
  Orbital Mechanics/1(v_ECI) -> Integrator/2  "V0"
  COE/1 -> Orbital Mechanics/1(COE)
  Constant/1 -> MATLAB Function1/2(mu)
  Constant1/1 -> Orbital Mechanics/2(mu)

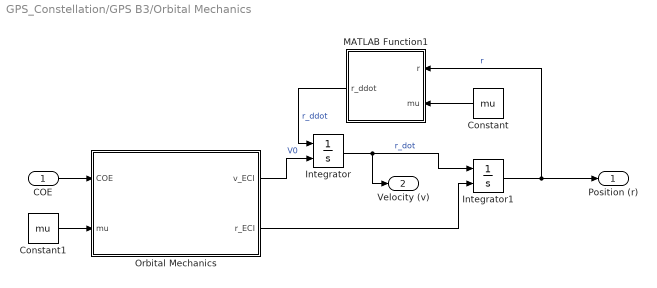
== system GPS_Constellation/GPS B3/Orbital Mechanics ==
  COE : Inport
  Constant : Constant  Value=mu
  Constant1 : Constant  Value=mu
  Integrator : Integrator  InitialConditionSource=external
  Integrator1 : Integrator  InitialConditionSource=external
  MATLAB Function1 : MATLAB Function  TreatAsAtomicUnit=on
  Orbital Mechanics : MATLAB Function  TreatAsAtomicUnit=on
  Position (r) : Outport
  Velocity (v) : Outport  Port=2
  wires:
  Integrator/1 -> Velocity (v)/1, Integrator1/1  "r_dot"
  MATLAB Function1/1(r_ddot) -> Integrator/1  "r_ddot"
  Integrator1/1 -> Position (r)/1, MATLAB Function1/1(r)  "r"
  Orbital Mechanics/2(r_ECI) -> Integrator1/2
  Orbital Mechanics/1(v_ECI) -> Integrator/2  "V0"
  COE/1 -> Orbital Mechanics/1(COE)
  Constant/1 -> MATLAB Function1/2(mu)
  Constant1/1 -> Orbital Mechanics/2(mu)

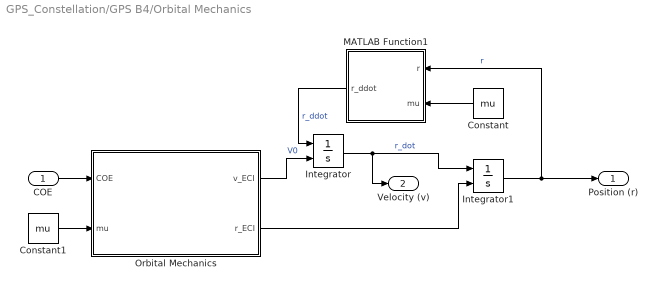
== system GPS_Constellation/GPS B4/Orbital Mechanics ==
  COE : Inport
  Constant : Constant  Value=mu
  Constant1 : Constant  Value=mu
  Integrator : Integrator  InitialConditionSource=external
  Integrator1 : Integrator  InitialConditionSource=external
  MATLAB Function1 : MATLAB Function  TreatAsAtomicUnit=on
  Orbital Mechanics : MATLAB Function  TreatAsAtomicUnit=on
  Position (r) : Outport
  Velocity (v) : Outport  Port=2
  wires:
  Integrator/1 -> Velocity (v)/1, Integrator1/1  "r_dot"
  MATLAB Function1/1(r_ddot) -> Integrator/1  "r_ddot"
  Integrator1/1 -> Position (r)/1, MATLAB Function1/1(r)  "r"
  Orbital Mechanics/2(r_ECI) -> Integrator1/2
  Orbital Mechanics/1(v_ECI) -> Integrator/2  "V0"
  COE/1 -> Orbital Mechanics/1(COE)
  Constant/1 -> MATLAB Function1/2(mu)
  Constant1/1 -> Orbital Mechanics/2(mu)

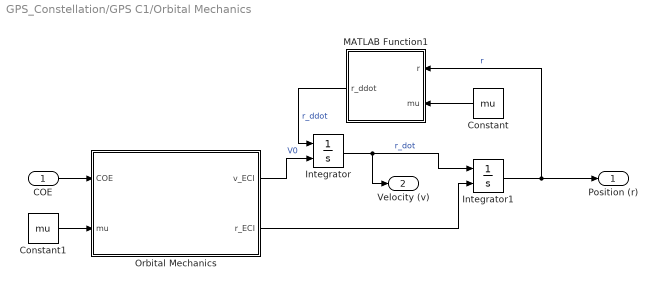
== system GPS_Constellation/GPS C1/Orbital Mechanics ==
  COE : Inport
  Constant : Constant  Value=mu
  Constant1 : Constant  Value=mu
  Integrator : Integrator  InitialConditionSource=external
  Integrator1 : Integrator  InitialConditionSource=external
  MATLAB Function1 : MATLAB Function  TreatAsAtomicUnit=on
  Orbital Mechanics : MATLAB Function  TreatAsAtomicUnit=on
  Position (r) : Outport
  Velocity (v) : Outport  Port=2
  wires:
  Integrator/1 -> Velocity (v)/1, Integrator1/1  "r_dot"
  MATLAB Function1/1(r_ddot) -> Integrator/1  "r_ddot"
  Integrator1/1 -> Position (r)/1, MATLAB Function1/1(r)  "r"
  Orbital Mechanics/2(r_ECI) -> Integrator1/2
  Orbital Mechanics/1(v_ECI) -> Integrator/2  "V0"
  COE/1 -> Orbital Mechanics/1(COE)
  Constant/1 -> MATLAB Function1/2(mu)
  Constant1/1 -> Orbital Mechanics/2(mu)

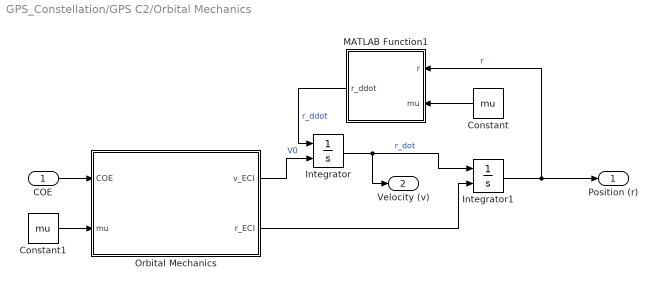
== system GPS_Constellation/GPS C2/Orbital Mechanics ==
  COE : Inport
  Constant : Constant  Value=mu
  Constant1 : Constant  Value=mu
  Integrator : Integrator  InitialConditionSource=external
  Integrator1 : Integrator  InitialConditionSource=external
  MATLAB Function1 : MATLAB Function  TreatAsAtomicUnit=on
  Orbital Mechanics : MATLAB Function  TreatAsAtomicUnit=on
  Position (r) : Outport
  Velocity (v) : Outport  Port=2
  wires:
  Integrator/1 -> Velocity (v)/1, Integrator1/1  "r_dot"
  MATLAB Function1/1(r_ddot) -> Integrator/1  "r_ddot"
  Integrator1/1 -> Position (r)/1, MATLAB Function1/1(r)  "r"
  Orbital Mechanics/2(r_ECI) -> Integrator1/2
  Orbital Mechanics/1(v_ECI) -> Integrator/2  "V0"
  COE/1 -> Orbital Mechanics/1(COE)
  Constant/1 -> MATLAB Function1/2(mu)
  Constant1/1 -> Orbital Mechanics/2(mu)

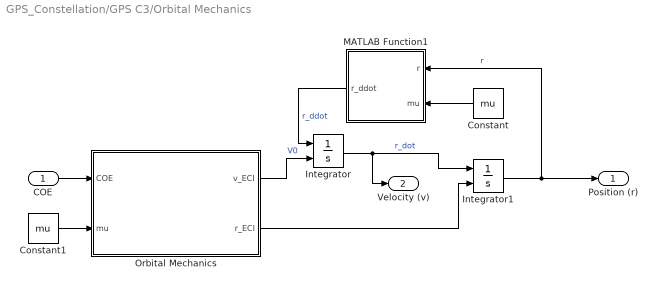
== system GPS_Constellation/GPS C3/Orbital Mechanics ==
  COE : Inport
  Constant : Constant  Value=mu
  Constant1 : Constant  Value=mu
  Integrator : Integrator  InitialConditionSource=external
  Integrator1 : Integrator  InitialConditionSource=external
  MATLAB Function1 : MATLAB Function  TreatAsAtomicUnit=on
  Orbital Mechanics : MATLAB Function  TreatAsAtomicUnit=on
  Position (r) : Outport
  Velocity (v) : Outport  Port=2
  wires:
  Integrator/1 -> Velocity (v)/1, Integrator1/1  "r_dot"
  MATLAB Function1/1(r_ddot) -> Integrator/1  "r_ddot"
  Integrator1/1 -> Position (r)/1, MATLAB Function1/1(r)  "r"
  Orbital Mechanics/2(r_ECI) -> Integrator1/2
  Orbital Mechanics/1(v_ECI) -> Integrator/2  "V0"
  COE/1 -> Orbital Mechanics/1(COE)
  Constant/1 -> MATLAB Function1/2(mu)
  Constant1/1 -> Orbital Mechanics/2(mu)

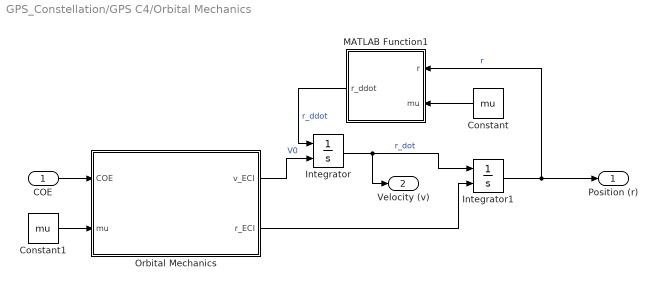
== system GPS_Constellation/GPS C4/Orbital Mechanics ==
  COE : Inport
  Constant : Constant  Value=mu
  Constant1 : Constant  Value=mu
  Integrator : Integrator  InitialConditionSource=external
  Integrator1 : Integrator  InitialConditionSource=external
  MATLAB Function1 : MATLAB Function  TreatAsAtomicUnit=on
  Orbital Mechanics : MATLAB Function  TreatAsAtomicUnit=on
  Position (r) : Outport
  Velocity (v) : Outport  Port=2
  wires:
  Integrator/1 -> Velocity (v)/1, Integrator1/1  "r_dot"
  MATLAB Function1/1(r_ddot) -> Integrator/1  "r_ddot"
  Integrator1/1 -> Position (r)/1, MATLAB Function1/1(r)  "r"
  Orbital Mechanics/2(r_ECI) -> Integrator1/2
  Orbital Mechanics/1(v_ECI) -> Integrator/2  "V0"
  COE/1 -> Orbital Mechanics/1(COE)
  Constant/1 -> MATLAB Function1/2(mu)
  Constant1/1 -> Orbital Mechanics/2(mu)

== system GPS_Constellation/GPS D1/Orbital Mechanics ==
  COE : Inport
  Constant : Constant  Value=mu
  Constant1 : Constant  Value=mu
  Integrator : Integrator  InitialConditionSource=external
  Integrator1 : Integrator  InitialConditionSource=external
  MATLAB Function1 : MATLAB Function  TreatAsAtomicUnit=on
  Orbital Mechanics : MATLAB Function  TreatAsAtomicUnit=on
  Position (r) : Outport
  Velocity (v) : Outport  Port=2
  wires:
  Integrator/1 -> Velocity (v)/1, Integrator1/1  "r_dot"
  MATLAB Function1/1(r_ddot) -> Integrator/1  "r_ddot"
  Integrator1/1 -> Position (r)/1, MATLAB Function1/1(r)  "r"
  Orbital Mechanics/2(r_ECI) -> Integrator1/2
  Orbital Mechanics/1(v_ECI) -> Integrator/2  "V0"
  COE/1 -> Orbital Mechanics/1(COE)
  Constant/1 -> MATLAB Function1/2(mu)
  Constant1/1 -> Orbital Mechanics/2(mu)

== system GPS_Constellation/GPS D2A/Orbital Mechanics ==
  COE : Inport
  Constant : Constant  Value=mu
  Constant1 : Constant  Value=mu
  Integrator : Integrator  InitialConditionSource=external
  Integrator1 : Integrator  InitialConditionSource=external
  MATLAB Function1 : MATLAB Function  TreatAsAtomicUnit=on
  Orbital Mechanics : MATLAB Function  TreatAsAtomicUnit=on
  Position (r) : Outport
  Velocity (v) : Outport  Port=2
  wires:
  Integrator/1 -> Velocity (v)/1, Integrator1/1  "r_dot"
  MATLAB Function1/1(r_ddot) -> Integrator/1  "r_ddot"
  Integrator1/1 -> Position (r)/1, MATLAB Function1/1(r)  "r"
  Orbital Mechanics/2(r_ECI) -> Integrator1/2
  Orbital Mechanics/1(v_ECI) -> Integrator/2  "V0"
  COE/1 -> Orbital Mechanics/1(COE)
  Constant/1 -> MATLAB Function1/2(mu)
  Constant1/1 -> Orbital Mechanics/2(mu)

== system GPS_Constellation/GPS D2F/Orbital Mechanics ==
  COE : Inport
  Constant : Constant  Value=mu
  Constant1 : Constant  Value=mu
  Integrator : Integrator  InitialConditionSource=external
  Integrator1 : Integrator  InitialConditionSource=external
  MATLAB Function1 : MATLAB Function  TreatAsAtomicUnit=on
  Orbital Mechanics : MATLAB Function  TreatAsAtomicUnit=on
  Position (r) : Outport
  Velocity (v) : Outport  Port=2
  wires:
  Integrator/1 -> Velocity (v)/1, Integrator1/1  "r_dot"
  MATLAB Function1/1(r_ddot) -> Integrator/1  "r_ddot"
  Integrator1/1 -> Position (r)/1, MATLAB Function1/1(r)  "r"
  Orbital Mechanics/2(r_ECI) -> Integrator1/2
  Orbital Mechanics/1(v_ECI) -> Integrator/2  "V0"
  COE/1 -> Orbital Mechanics/1(COE)
  Constant/1 -> MATLAB Function1/2(mu)
  Constant1/1 -> Orbital Mechanics/2(mu)

== system GPS_Constellation/GPS D3/Orbital Mechanics ==
  COE : Inport
  Constant : Constant  Value=mu
  Constant1 : Constant  Value=mu
  Integrator : Integrator  InitialConditionSource=external
  Integrator1 : Integrator  InitialConditionSource=external
  MATLAB Function1 : MATLAB Function  TreatAsAtomicUnit=on
  Orbital Mechanics : MATLAB Function  TreatAsAtomicUnit=on
  Position (r) : Outport
  Velocity (v) : Outport  Port=2
  wires:
  Integrator/1 -> Velocity (v)/1, Integrator1/1  "r_dot"
  MATLAB Function1/1(r_ddot) -> Integrator/1  "r_ddot"
  Integrator1/1 -> Position (r)/1, MATLAB Function1/1(r)  "r"
  Orbital Mechanics/2(r_ECI) -> Integrator1/2
  Orbital Mechanics/1(v_ECI) -> Integrator/2  "V0"
  COE/1 -> Orbital Mechanics/1(COE)
  Constant/1 -> MATLAB Function1/2(mu)
  Constant1/1 -> Orbital Mechanics/2(mu)

== system GPS_Constellation/GPS D4/Orbital Mechanics ==
  COE : Inport
  Constant : Constant  Value=mu
  Constant1 : Constant  Value=mu
  Integrator : Integrator  InitialConditionSource=external
  Integrator1 : Integrator  InitialConditionSource=external
  MATLAB Function1 : MATLAB Function  TreatAsAtomicUnit=on
  Orbital Mechanics : MATLAB Function  TreatAsAtomicUnit=on
  Position (r) : Outport
  Velocity (v) : Outport  Port=2
  wires:
  Integrator/1 -> Velocity (v)/1, Integrator1/1  "r_dot"
  MATLAB Function1/1(r_ddot) -> Integrator/1  "r_ddot"
  Integrator1/1 -> Position (r)/1, MATLAB Function1/1(r)  "r"
  Orbital Mechanics/2(r_ECI) -> Integrator1/2
  Orbital Mechanics/1(v_ECI) -> Integrator/2  "V0"
  COE/1 -> Orbital Mechanics/1(COE)
  Constant/1 -> MATLAB Function1/2(mu)
  Constant1/1 -> Orbital Mechanics/2(mu)

== system GPS_Constellation/GPS E1/Orbital Mechanics ==
  COE : Inport
  Constant : Constant  Value=mu
  Constant1 : Constant  Value=mu
  Integrator : Integrator  InitialConditionSource=external
  Integrator1 : Integrator  InitialConditionSource=external
  MATLAB Function1 : MATLAB Function  TreatAsAtomicUnit=on
  Orbital Mechanics : MATLAB Function  TreatAsAtomicUnit=on
  Position (r) : Outport
  Velocity (v) : Outport  Port=2
  wires:
  Integrator/1 -> Velocity (v)/1, Integrator1/1  "r_dot"
  MATLAB Function1/1(r_ddot) -> Integrator/1  "r_ddot"
  Integrator1/1 -> Position (r)/1, MATLAB Function1/1(r)  "r"
  Orbital Mechanics/2(r_ECI) -> Integrator1/2
  Orbital Mechanics/1(v_ECI) -> Integrator/2  "V0"
  COE/1 -> Orbital Mechanics/1(COE)
  Constant/1 -> MATLAB Function1/2(mu)
  Constant1/1 -> Orbital Mechanics/2(mu)

== system GPS_Constellation/GPS E2/Orbital Mechanics ==
  COE : Inport
  Constant : Constant  Value=mu
  Constant1 : Constant  Value=mu
  Integrator : Integrator  InitialConditionSource=external
  Integrator1 : Integrator  InitialConditionSource=external
  MATLAB Function1 : MATLAB Function  TreatAsAtomicUnit=on
  Orbital Mechanics : MATLAB Function  TreatAsAtomicUnit=on
  Position (r) : Outport
  Velocity (v) : Outport  Port=2
  wires:
  Integrator/1 -> Velocity (v)/1, Integrator1/1  "r_dot"
  MATLAB Function1/1(r_ddot) -> Integrator/1  "r_ddot"
  Integrator1/1 -> Position (r)/1, MATLAB Function1/1(r)  "r"
  Orbital Mechanics/2(r_ECI) -> Integrator1/2
  Orbital Mechanics/1(v_ECI) -> Integrator/2  "V0"
  COE/1 -> Orbital Mechanics/1(COE)
  Constant/1 -> MATLAB Function1/2(mu)
  Constant1/1 -> Orbital Mechanics/2(mu)

== system GPS_Constellation/GPS E3/Orbital Mechanics ==
  COE : Inport
  Constant : Constant  Value=mu
  Constant1 : Constant  Value=mu
  Integrator : Integrator  InitialConditionSource=external
  Integrator1 : Integrator  InitialConditionSource=external
  MATLAB Function1 : MATLAB Function  TreatAsAtomicUnit=on
  Orbital Mechanics : MATLAB Function  TreatAsAtomicUnit=on
  Position (r) : Outport
  Velocity (v) : Outport  Port=2
  wires:
  Integrator/1 -> Velocity (v)/1, Integrator1/1  "r_dot"
  MATLAB Function1/1(r_ddot) -> Integrator/1  "r_ddot"
  Integrator1/1 -> Position (r)/1, MATLAB Function1/1(r)  "r"
  Orbital Mechanics/2(r_ECI) -> Integrator1/2
  Orbital Mechanics/1(v_ECI) -> Integrator/2  "V0"
  COE/1 -> Orbital Mechanics/1(COE)
  Constant/1 -> MATLAB Function1/2(mu)
  Constant1/1 -> Orbital Mechanics/2(mu)

== system GPS_Constellation/GPS E4/Orbital Mechanics ==
  COE : Inport
  Constant : Constant  Value=mu
  Constant1 : Constant  Value=mu
  Integrator : Integrator  InitialConditionSource=external
  Integrator1 : Integrator  InitialConditionSource=external
  MATLAB Function1 : MATLAB Function  TreatAsAtomicUnit=on
  Orbital Mechanics : MATLAB Function  TreatAsAtomicUnit=on
  Position (r) : Outport
  Velocity (v) : Outport  Port=2
  wires:
  Integrator/1 -> Velocity (v)/1, Integrator1/1  "r_dot"
  MATLAB Function1/1(r_ddot) -> Integrator/1  "r_ddot"
  Integrator1/1 -> Position (r)/1, MATLAB Function1/1(r)  "r"
  Orbital Mechanics/2(r_ECI) -> Integrator1/2
  Orbital Mechanics/1(v_ECI) -> Integrator/2  "V0"
  COE/1 -> Orbital Mechanics/1(COE)
  Constant/1 -> MATLAB Function1/2(mu)
  Constant1/1 -> Orbital Mechanics/2(mu)

== system GPS_Constellation/GPS F1/Orbital Mechanics ==
  COE : Inport
  Constant : Constant  Value=mu
  Constant1 : Constant  Value=mu
  Integrator : Integrator  InitialConditionSource=external
  Integrator1 : Integrator  InitialConditionSource=external
  MATLAB Function1 : MATLAB Function  TreatAsAtomicUnit=on
  Orbital Mechanics : MATLAB Function  TreatAsAtomicUnit=on
  Position (r) : Outport
  Velocity (v) : Outport  Port=2
  wires:
  Integrator/1 -> Velocity (v)/1, Integrator1/1  "r_dot"
  MATLAB Function1/1(r_ddot) -> Integrator/1  "r_ddot"
  Integrator1/1 -> Position (r)/1, MATLAB Function1/1(r)  "r"
  Orbital Mechanics/2(r_ECI) -> Integrator1/2
  Orbital Mechanics/1(v_ECI) -> Integrator/2  "V0"
  COE/1 -> Orbital Mechanics/1(COE)
  Constant/1 -> MATLAB Function1/2(mu)
  Constant1/1 -> Orbital Mechanics/2(mu)

== system GPS_Constellation/GPS F2A/Orbital Mechanics ==
  COE : Inport
  Constant : Constant  Value=mu
  Constant1 : Constant  Value=mu
  Integrator : Integrator  InitialConditionSource=external
  Integrator1 : Integrator  InitialConditionSource=external
  MATLAB Function1 : MATLAB Function  TreatAsAtomicUnit=on
  Orbital Mechanics : MATLAB Function  TreatAsAtomicUnit=on
  Position (r) : Outport
  Velocity (v) : Outport  Port=2
  wires:
  Integrator/1 -> Velocity (v)/1, Integrator1/1  "r_dot"
  MATLAB Function1/1(r_ddot) -> Integrator/1  "r_ddot"
  Integrator1/1 -> Position (r)/1, MATLAB Function1/1(r)  "r"
  Orbital Mechanics/2(r_ECI) -> Integrator1/2
  Orbital Mechanics/1(v_ECI) -> Integrator/2  "V0"
  COE/1 -> Orbital Mechanics/1(COE)
  Constant/1 -> MATLAB Function1/2(mu)
  Constant1/1 -> Orbital Mechanics/2(mu)

== system GPS_Constellation/GPS F2F/Orbital Mechanics ==
  COE : Inport
  Constant : Constant  Value=mu
  Constant1 : Constant  Value=mu
  Integrator : Integrator  InitialConditionSource=external
  Integrator1 : Integrator  InitialConditionSource=external
  MATLAB Function1 : MATLAB Function  TreatAsAtomicUnit=on
  Orbital Mechanics : MATLAB Function  TreatAsAtomicUnit=on
  Position (r) : Outport
  Velocity (v) : Outport  Port=2
  wires:
  Integrator/1 -> Velocity (v)/1, Integrator1/1  "r_dot"
  MATLAB Function1/1(r_ddot) -> Integrator/1  "r_ddot"
  Integrator1/1 -> Position (r)/1, MATLAB Function1/1(r)  "r"
  Orbital Mechanics/2(r_ECI) -> Integrator1/2
  Orbital Mechanics/1(v_ECI) -> Integrator/2  "V0"
  COE/1 -> Orbital Mechanics/1(COE)
  Constant/1 -> MATLAB Function1/2(mu)
  Constant1/1 -> Orbital Mechanics/2(mu)

== system GPS_Constellation/GPS F3/Orbital Mechanics ==
  COE : Inport
  Constant : Constant  Value=mu
  Constant1 : Constant  Value=mu
  Integrator : Integrator  InitialConditionSource=external
  Integrator1 : Integrator  InitialConditionSource=external
  MATLAB Function1 : MATLAB Function  TreatAsAtomicUnit=on
  Orbital Mechanics : MATLAB Function  TreatAsAtomicUnit=on
  Position (r) : Outport
  Velocity (v) : Outport  Port=2
  wires:
  Integrator/1 -> Velocity (v)/1, Integrator1/1  "r_dot"
  MATLAB Function1/1(r_ddot) -> Integrator/1  "r_ddot"
  Integrator1/1 -> Position (r)/1, MATLAB Function1/1(r)  "r"
  Orbital Mechanics/2(r_ECI) -> Integrator1/2
  Orbital Mechanics/1(v_ECI) -> Integrator/2  "V0"
  COE/1 -> Orbital Mechanics/1(COE)
  Constant/1 -> MATLAB Function1/2(mu)
  Constant1/1 -> Orbital Mechanics/2(mu)

== system GPS_Constellation/GPS F4/Orbital Mechanics ==
  COE : Inport
  Constant : Constant  Value=mu
  Constant1 : Constant  Value=mu
  Integrator : Integrator  InitialConditionSource=external
  Integrator1 : Integrator  InitialConditionSource=external
  MATLAB Function1 : MATLAB Function  TreatAsAtomicUnit=on
  Orbital Mechanics : MATLAB Function  TreatAsAtomicUnit=on
  Position (r) : Outport
  Velocity (v) : Outport  Port=2
  wires:
  Integrator/1 -> Velocity (v)/1, Integrator1/1  "r_dot"
  MATLAB Function1/1(r_ddot) -> Integrator/1  "r_ddot"
  Integrator1/1 -> Position (r)/1, MATLAB Function1/1(r)  "r"
  Orbital Mechanics/2(r_ECI) -> Integrator1/2
  Orbital Mechanics/1(v_ECI) -> Integrator/2  "V0"
  COE/1 -> Orbital Mechanics/1(COE)
  Constant/1 -> MATLAB Function1/2(mu)
  Constant1/1 -> Orbital Mechanics/2(mu)

== matlab function GPS_Constellation/GPS A1 /Orbital Mechanics/MATLAB Function1 ==
  data: R_sat input; r_ddot output; mu parameter
function r_ddot = r_ddot(R_sat, mu)
% ========================================================================
% Description: This function calculates the accelerations acting on the
% spacecraft body

r_ddot = -(mu/(norm(R_sat))^3)*R_sat;

end
% ========================================================================
